simulink model "sf_msg_basic_semantics"  (R2017b)
settings: Solver=FixedStepDiscrete  StartTime=0.0  StopTime=10.0  FixedStep=1  RelTol=1e-3  EnableMultiTasking=on
settings Model: Creator=The MathWorks, Inc.  LastModifiedBy=The MathWorks, Inc.
settings DataIOCC: LimitDataPoints=on  SaveFormat=Array
settings OptimizationCC: ExpressionDepthLimit=2147483647  LifeSpan=1
settings DebuggingCC: UnderspecifiedInitializationDetection=Classic  MergeDetectMultiDrivingBlocksExec=none  SolverPrmCheckMsg=warning  AllowSymbolicDim=off  StateNameClashWarn=warning  SFUnexpectedBacktrackingDiag=warning  SFNoUnconditionalDefaultTransitionDiag=warning  SFExecutionAtInitializationDiag=none
settings HardwareCC: ProdBitPerPointer=32  ProdBitPerSizeT=32  ProdBitPerPtrDiffT=32  ProdLargestAtomicFloat=None  ProdIntDivRoundTo=Undefined  ProdEndianess=Unspecified  ProdWordSize=32  ProdHWDeviceType=32-bit Generic
settings ModelReferenceCC: PropagateSignalLabelsOutOfModel=off
settings SFSimCC: MATLABDynamicMemAlloc=off
settings RTWCC: SystemTargetFile=ert.tlc  TemplateMakefile=ert_default_tmf  Description=Real-Time Workshop Embedded Coder
settings CodeAppCC: IgnoreCustomStorageClasses=off  CustomSymbolStrType=$N$R$M  StateflowObjectComments=on  InternalIdentifier=Classic
settings ERTTargetCC: MultiwordLength=2048  GenerateSampleERTMain=on  ERTCustomFileTemplate=example_file_process.tlc  ConvertIfToSwitch=off  SuppressUnreachableDefaultCases=off
settings ConfigComp: CovMetricSettings=dw  CovHtmlReporting=on  CovSaveCumulativeToWorkspaceVar=on  CovSaveSingleToWorkspaceVar=on  CovExternalEMLEnable=off  CovSFcnEnable=off

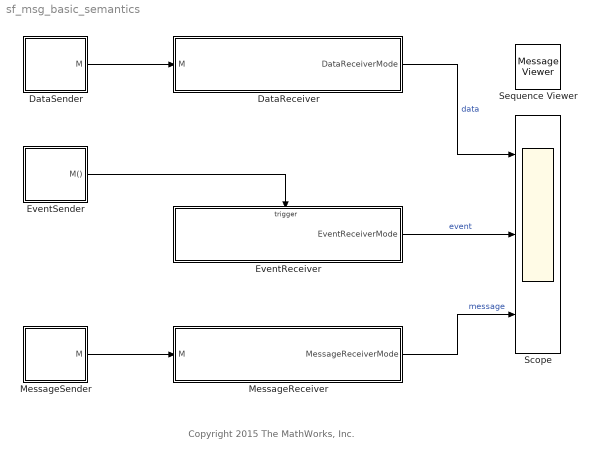
== system sf_msg_basic_semantics ==
  note: Copyright 2015 The MathWorks, Inc.
  DataReceiver : Stateflow chart  TreatAsAtomicUnit=on
  DataSender : Stateflow chart  TreatAsAtomicUnit=on
  EventReceiver : Stateflow chart  TreatAsAtomicUnit=on
  EventSender : Stateflow chart  TreatAsAtomicUnit=on
  MessageReceiver : Stateflow chart  TreatAsAtomicUnit=on
  MessageSender : Stateflow chart  TreatAsAtomicUnit=on
  Scope : Scope  NumInputPorts=3
  Sequence Viewer : MessageViewer
  wires:
  MessageSender/1(M) -> MessageReceiver/1(M)
  EventSender/1(M()) -> EventReceiver/Trigger
  DataSender/1(M) -> DataReceiver/1(M)
  EventReceiver/1(EventReceiverMode) -> Scope/2  "event"
  MessageReceiver/1(MessageReceiverMode) -> Scope/3  "message"
  DataReceiver/1(DataReceiverMode) -> Scope/1  "data"

== stateflow chart sf_msg_basic_semantics/MessageSender ==
  state A
    en:
    send(M);
  (default) -> A
  data: M output double

== stateflow chart sf_msg_basic_semantics/MessageReceiver ==
  state A0
  state A1
  state A2
  state A3
  (default) -> A0
  A0 -> A1 : after(3,sec)
  A1 -> A2 : M
  A2 -> A3 : M
  data: M input double; MessageReceiverMode output Enum: MessageReceiverModeType

== stateflow chart sf_msg_basic_semantics/EventReceiver ==
  state A0
  state A1
  state A2
  state A3
  (default) -> A0
  A0 -> A1 : after(3,sec)
  A1 -> A2 : M
  A2 -> A3 : M
  data: EventReceiverMode output Enum: EventReceiverModeType
  events: M input FUNCTION_CALL_EVENT

== stateflow chart sf_msg_basic_semantics/EventSender ==
  state A
    en: send(M)
  (default) -> A
  events: M output FUNCTION_CALL_EVENT

== stateflow chart sf_msg_basic_semantics/DataReceiver ==
  state A0
  state A1
  state A2
  state A3
  (default) -> A0
  A0 -> A1 : after(3,sec)
  A1 -> A2 : [M == 1]
  A2 -> A3 : [M == 1]
  data: M input double; DataReceiverMode output Enum: DataReceiverModeType

== stateflow chart sf_msg_basic_semantics/DataSender ==
  state A
    en: M = 1;
  (default) -> A
  data: M output double
